simulink model "Testbench_for_Power_Circulating_TopologyB"  (R2023b)
settings: Solver=VariableStepAuto  StartTime=0.0  StopTime=1  RelTol=1e-3
InitFcn:
  | Initialization_for_Testbench;
values from neighbouring files (symbols this model uses):
  Cdc = 180e-6    (= 0.00018)    [CurrentLoop.m]    (also in Initialization_for_ESS_3P_2L_220kW.m; Initialization_for_Testbench.m)
  Fnom_Grid = 50    [CurrentLoop.m]    (also in Initialization_for_ESS_3P_2L_220kW.m; Initialization_for_Testbench.m)
  Inom = Pnom/sqrt(3)/Unom_Grid    [CurrentLoop.m]    (also in Initialization_for_ESS_3P_2L_220kW.m; Initialization_for_Testbench.m)
  Ki_Idq = Kp_Idq*2*pi*2    (= 40.2123859659)    [Initialization_for_ESS_3P_2L_220kW.m]    (also in Initialization_for_Testbench.m = 1.26330936334)
  Kp_Idq = L_grid/3/Ts_Control*3    (= 3.2)    [Initialization_for_ESS_3P_2L_220kW.m]    (also in Initialization_for_Testbench.m = 2.0106192983)
  L_grid = 200e-6    (= 0.0002)    [Initialization_for_ESS_3P_2L_220kW.m]    (also in Initialization_for_Testbench.m)
  Pnom = 220e3    (= 220000)    [CurrentLoop.m]    (also in Initialization_for_ESS_3P_2L_220kW.m; Initialization_for_Testbench.m = 2500000)
  Ts_Control = 62.5e-6    (= 6.25e-05)    [CurrentLoop.m]    (also in Initialization_for_ESS_3P_2L_220kW.m; Initialization_for_Testbench.m = 0.0001)
  Ts_Power = 10e-7    (= 1e-06)    [Initialization_for_ESS_3P_2L_220kW.m]    (also in Initialization_for_Testbench.m)
  Udc_ref = 1500    [CurrentLoop.m]    (also in Initialization_for_ESS_3P_2L_220kW.m; Initialization_for_Testbench.m)
  Unom_Phase = Unom_Grid/sqrt(3)    [CurrentLoop.m]    (also in Initialization_for_ESS_3P_2L_220kW.m; Initialization_for_Testbench.m)
libraries: LibraryForCodeGeneration x10, spsSeriesRLCBranchLib x4, spsTriangleGeneratorLib x2, spsUniversalBridgeLib x2, spsCurrentMeasurementLib x1, spsDCVoltageSourceLib x1, spsStairGeneratorLib x1, spsThreePhaseSeriesRLCBranchLib x1, spsThreePhaseVIMeasurementLib x1, spsVoltageMeasurementLib x1, spspowerguiLib x1
settings Model: DataDictionary=VariablesDictionary_for_Testbench_TopologyB.sldd  Creator=ZZY  LastModifiedBy=ZZY

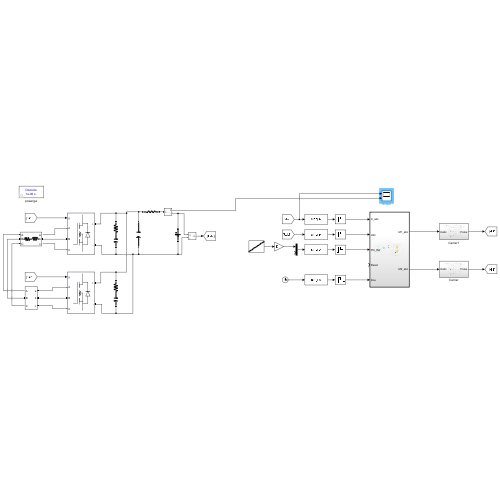
[thumbnail: Simulink's stored preview of the top-level diagram]
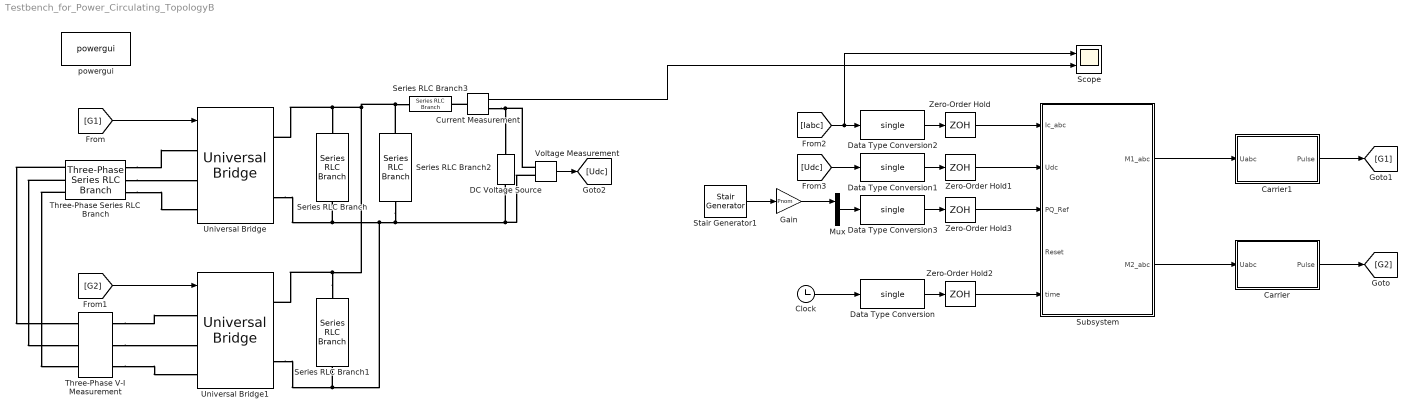
== system Testbench_for_Power_Circulating_TopologyB ==
  Carrier : Subsystem
  Carrier1 : Subsystem
  Clock : Clock
  Current Measurement : spsCurrentMeasurementLib/Current Measurement  PhasorSimulation=off  OutputType=Complex  PSBequivalent=0
  DC Voltage Source : spsDCVoltageSourceLib/DC Voltage Source  Amplitude=Udc_ref  Measurements=None
  Data Type Conversion{,1..3} (4 alike) : DataTypeConversion  OutDataTypeStr=single  SaturateOnIntegerOverflow=off  RndMeth=Floor
  Gain : Gain  Gain=Pnom
  Mux : Mux  Inputs=2
  Scope : Scope  NumInputPorts=2
  Series RLC Branch : spsSeriesRLCBranchLib/Series RLC Branch  LConnTagsString=__new0  RConnTagsString=__new0  BranchType=RC  Resistance=1e-6  Inductance=1e-3  SetiL0=off  InitialCurrent=0  Capacitance=Cdc  Setx0=on  InitialVoltage=Udc_ref  Measurements=Branch voltage
  Series RLC Branch1 : spsSeriesRLCBranchLib/Series RLC Branch  LConnTagsString=__new0  RConnTagsString=__new0  BranchType=RC  Resistance=1e-6  Inductance=1e-3  SetiL0=off  InitialCurrent=0  Capacitance=Cdc  Setx0=on  InitialVoltage=Udc_ref  Measurements=Branch voltage
  Series RLC Branch2 : spsSeriesRLCBranchLib/Series RLC Branch  LConnTagsString=__new0  RConnTagsString=__new0  BranchType=C  Resistance=1e-6  Inductance=1e-3  SetiL0=off  InitialCurrent=0  Capacitance=Cdc*100  Setx0=on  InitialVoltage=Udc_ref  Measurements=Branch voltage
  Series RLC Branch3 : spsSeriesRLCBranchLib/Series RLC Branch  LConnTagsString=__new0  RConnTagsString=__new0  BranchType=R  Resistance=1e-2  Inductance=1e-3  SetiL0=off  InitialCurrent=0  Capacitance=Cdc*100  Setx0=on  InitialVoltage=Udc_ref  Measurements=Branch voltage
  Stair Generator1 : spsStairGeneratorLib/Stair Generator  t=0:0.1:1  e=0:0.1:1  Ts=0
  Subsystem : Subsystem  TreatAsAtomicUnit=on  SystemSampleTime=Ts_Control
  Three-Phase Series RLC Branch : spsThreePhaseSeriesRLCBranchLib/Three-Phase Series RLC Branch  LConnTagsString=A|B|C  RConnTagsString=A|B|C  BranchType=RL  Resistance=1e-3  Inductance=L_grid*1  Capacitance=1e-6  Measurements=None
  Three-Phase V-I Measurement : spsThreePhaseVIMeasurementLib/Three-Phase V-I Measurement  VoltageMeasurement=no  SetLabelV=off  LabelV=Vabc  Vpu=off  VpuLL=off  CurrentMeasurement=yes  SetLabelI=on  LabelI=Iabc  Ipu=off  Pbase=100e6  Vbase=500e3  OutputType=Complex  PhasorSimulation=off  PSBequivalent=0
  Universal Bridge : spsUniversalBridgeLib/Universal Bridge  Arms=3  SnubberResistance=1e5  SnubberCapacitance=inf  Device=MOSFET / Diodes  Ron=1e-3  Lon=0  ForwardVoltages="[  0  0  ]"  ForwardVoltage=0  GTOparameters=[ 10e-6 , 20e-6 ]  IGBTparameters=[ 1e-6 , 2e-6 ]  Measurements=None  Measurements_2=None  converterType=Rectifier
  Universal Bridge1 : spsUniversalBridgeLib/Universal Bridge  Arms=3  SnubberResistance=1e5  SnubberCapacitance=inf  Device=MOSFET / Diodes  Ron=1e-3  Lon=0  ForwardVoltages="[  0  0  ]"  ForwardVoltage=0  GTOparameters=[ 10e-6 , 20e-6 ]  IGBTparameters=[ 1e-6 , 2e-6 ]  Measurements=None  Measurements_2=None  converterType=Rectifier
  Voltage Measurement : spsVoltageMeasurementLib/Voltage Measurement  PhasorSimulation=off  OutputType=Complex  PSBequivalent=0
  Zero-Order Hold{,1..3} (4 alike) : ZeroOrderHold  SampleTime=Ts_Control
  powergui : spspowerguiLib/powergui  Priority=1  SimulationMode=Discrete  SampleTime=Ts_Power  frequency=60  Iterations=50  frequencyindice=0  Pbase=100e6  ErrMax=1e-4  UnitsV=kV  UnitsW=MW  buscounter=0  FunctionMessages=off  echomessages=off  EnableUseOfTLC=off  CurrentSourceSwitches=off  DisableSnubberDevices=off  DisableRonSwitches=off  DisableVfSwitches=off  DisplayEquations=off  AutomaticDiscreteSolvers=off  SolverType=Tustin/Backward Euler (TBE)  Interpol=off  ExternalGateDelay=off  methode=off  Ts=100  x0status=blocks  SPID=on  SwTol=0  HookPort=off  NonlinearTolerance=1e-4  nMaxIteration=100  ContinueOnMaxIteration=off  RestoreLinks=warning  ResistiveCurrentMeasurement=off  Frange=[0:2:500]  Ylog=off  Xlog=on  ShowGrid=off  save=off  variable=ZData  structure=CHB_abc  ZoomFFT=off  StartTime=1.4  cycles=5  DisplayStyle=1  fundamental=50  FreqAxis=off  MaxFrequency=30000  frequencyindicesteady=1  RmsSteady=1  display=off
  wires:
  Subsystem/2(M2_abc) -> Carrier/1(Uabc)
  Carrier/1(Pulse) -> [G2]
  Carrier1/1(Pulse) -> [G1]
  Subsystem/1(M1_abc) -> Carrier1/1(Uabc)
  [G1] -> Universal Bridge/1
  [Iabc] -> Scope/1, Data Type Conversion2/1
  [G2] -> Universal Bridge1/1
  Zero-Order Hold/1 -> Subsystem/1(Ic_abc)
  Voltage Measurement/1 -> [Udc]
  [Udc] -> Data Type Conversion1/1
  Zero-Order Hold1/1 -> Subsystem/2(Udc)
  Clock/1 -> Data Type Conversion/1
  Zero-Order Hold2/1 -> Subsystem/5(time)
  Data Type Conversion/1 -> Zero-Order Hold2/1
  Data Type Conversion1/1 -> Zero-Order Hold1/1
  Data Type Conversion2/1 -> Zero-Order Hold/1
  Data Type Conversion3/1 -> Zero-Order Hold3/1
  Zero-Order Hold3/1 -> Subsystem/3(PQ_Ref)
  Mux/1 -> Data Type Conversion3/1
  Stair Generator1/1 -> Gain/1
  Gain/1 -> Mux/1
  Current Measurement/1 -> Scope/2
  connections:
  Series RLC Branch1/LConn1 -- Series RLC Branch3/RConn1 -- Series RLC Branch2/LConn1 -- Universal Bridge/RConn1 -- Series RLC Branch/LConn1 -- Universal Bridge1/RConn1
  Series RLC Branch1/RConn1 -- Voltage Measurement/LConn2 -- DC Voltage Source/LConn1 -- Series RLC Branch2/RConn1 -- Universal Bridge/RConn2 -- Series RLC Branch/RConn1 -- Universal Bridge1/RConn2
  Three-Phase Series RLC Branch/RConn2 -- Universal Bridge/LConn2
  Three-Phase Series RLC Branch/RConn1 -- Universal Bridge/LConn1
  Three-Phase Series RLC Branch/RConn3 -- Universal Bridge/LConn3
  Three-Phase Series RLC Branch/LConn3 -- Three-Phase V-I Measurement/LConn3
  Three-Phase Series RLC Branch/LConn2 -- Three-Phase V-I Measurement/LConn2
  Three-Phase Series RLC Branch/LConn1 -- Three-Phase V-I Measurement/LConn1
  Three-Phase V-I Measurement/RConn1 -- Universal Bridge1/LConn1
  Three-Phase V-I Measurement/RConn2 -- Universal Bridge1/LConn2
  Three-Phase V-I Measurement/RConn3 -- Universal Bridge1/LConn3
  Voltage Measurement/LConn1 -- Current Measurement/RConn1 -- DC Voltage Source/RConn1
  Current Measurement/LConn1 -- Series RLC Branch3/LConn1

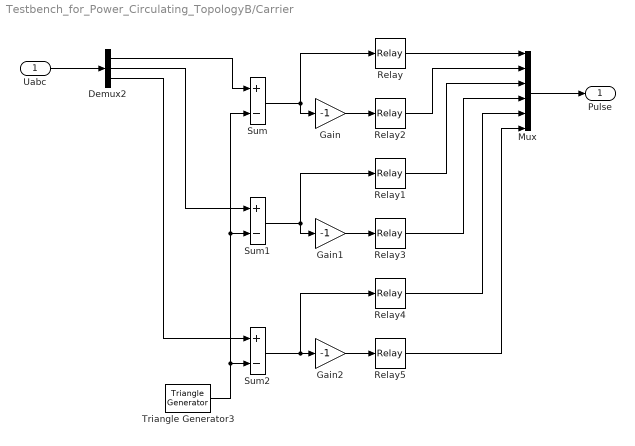
== system Testbench_for_Power_Circulating_TopologyB/Carrier ==
  Uabc : Inport
  Demux2 : Demux  Outputs=3
  Gain : Gain  Gain=-1
  Gain1 : Gain  Gain=-1
  Gain2 : Gain  Gain=-1
  Mux : Mux  Inputs=6
  Relay{,1..5} (6 alike) : Relay  OffSwitchValue=-eps
  Sum : Sum  Inputs=+-
  Sum1 : Sum  Inputs=+-
  Sum2 : Sum  Inputs=+-
  Triangle Generator3 : spsTriangleGeneratorLib/Triangle Generator  Freq=Fsw  Phase=180  Ts=Ts_Power
  Pulse : Outport
  wires:
  Mux/1 -> Pulse/1
  Gain/1 -> Relay2/1
  Sum/1 -> Relay/1, Gain/1
  Uabc/1 -> Demux2/1
  Demux2/1 -> Sum/1
  Relay/1 -> Mux/1
  Relay2/1 -> Mux/2
  Relay1/1 -> Mux/3
  Relay3/1 -> Mux/4
  Gain1/1 -> Relay3/1
  Demux2/2 -> Sum1/1
  Sum1/1 -> Relay1/1, Gain1/1
  Relay5/1 -> Mux/6
  Demux2/3 -> Sum2/1
  Gain2/1 -> Relay5/1
  Sum2/1 -> Relay4/1, Gain2/1
  Relay4/1 -> Mux/5
  Triangle Generator3/1 -> Sum/2, Sum1/2, Sum2/2

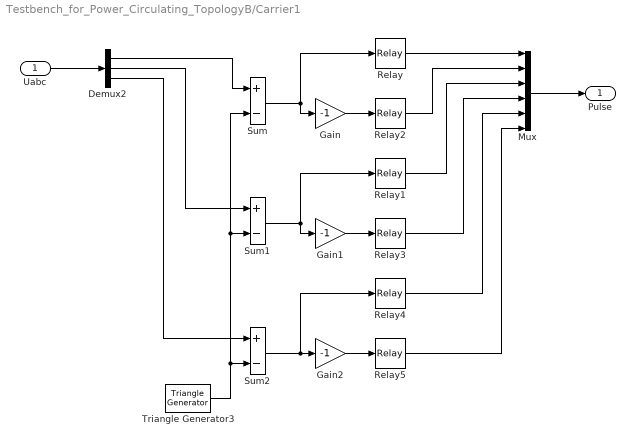
== system Testbench_for_Power_Circulating_TopologyB/Carrier1 ==
  Uabc : Inport
  Demux2 : Demux  Outputs=3
  Gain : Gain  Gain=-1
  Gain1 : Gain  Gain=-1
  Gain2 : Gain  Gain=-1
  Mux : Mux  Inputs=6
  Relay{,1..5} (6 alike) : Relay  OffSwitchValue=-eps
  Sum : Sum  Inputs=+-
  Sum1 : Sum  Inputs=+-
  Sum2 : Sum  Inputs=+-
  Triangle Generator3 : spsTriangleGeneratorLib/Triangle Generator  Freq=Fsw  Phase=180  Ts=Ts_Power
  Pulse : Outport
  wires:
  Mux/1 -> Pulse/1
  Gain/1 -> Relay2/1
  Sum/1 -> Relay/1, Gain/1
  Uabc/1 -> Demux2/1
  Demux2/1 -> Sum/1
  Relay/1 -> Mux/1
  Relay2/1 -> Mux/2
  Relay1/1 -> Mux/3
  Relay3/1 -> Mux/4
  Gain1/1 -> Relay3/1
  Demux2/2 -> Sum1/1
  Sum1/1 -> Relay1/1, Gain1/1
  Relay5/1 -> Mux/6
  Demux2/3 -> Sum2/1
  Gain2/1 -> Relay5/1
  Sum2/1 -> Relay4/1, Gain2/1
  Relay4/1 -> Mux/5
  Triangle Generator3/1 -> Sum/2, Sum1/2, Sum2/2

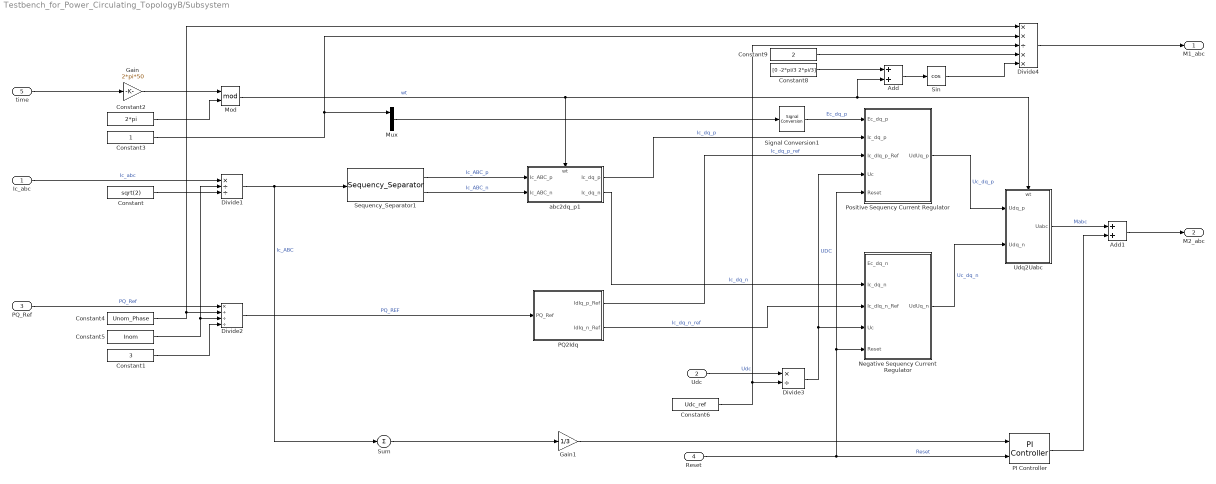
== system Testbench_for_Power_Circulating_TopologyB/Subsystem ==
  Ic_abc : Inport  OutDataTypeStr=single
  Udc : Inport  Port=2  OutDataTypeStr=single
  PQ_Ref : Inport  Port=3  OutDataTypeStr=single
  Reset : Inport  Port=4  OutDataTypeStr=boolean
  time : Inport  Port=5  OutDataTypeStr=single
  Add : Sum
  Add1 : Sum
  Constant : Constant  Value=sqrt(2)  OutDataTypeStr=single  SampleTime=-1
  Constant1 : Constant  Value=3  OutDataTypeStr=Inherit: Inherit via back propagation  SampleTime=-1
  Constant2 : Constant  Value=2*pi  OutDataTypeStr=single  SampleTime=-1
  Constant3 : Constant  OutDataTypeStr=single  SampleTime=-1
  Constant4 : Constant  Value=Unom_Phase  OutDataTypeStr=Inherit: Inherit via back propagation  SampleTime=-1
  Constant5 : Constant  Value=Inom  OutDataTypeStr=Inherit: Inherit via back propagation  SampleTime=-1
  Constant6 : Constant  Value=Udc_ref  OutDataTypeStr=Inherit: Inherit via back propagation  SampleTime=-1
  Constant8 : Constant  Value=[0 -2*pi/3 2*pi/3]  OutDataTypeStr=Inherit: Inherit via back propagation  SampleTime=-1
  Constant9 : Constant  Value=2  OutDataTypeStr=Inherit: Inherit via back propagation  SampleTime=-1
  Divide1 : Product  Inputs=*//  OutDataTypeStr=single
  Divide2 : Product  Inputs=*///  OutDataTypeStr=single
  Divide3 : Product  Inputs=*/  OutDataTypeStr=single
  Divide4 : Product  Inputs=**/**  OutDataTypeStr=single
  Gain : Gain  Gain=2*pi*50
  Gain1 : Gain  Gain=1/3
  Mod : Math  Operator=mod
  Mux : Mux  Inputs=2
  Negative Sequency Current Regulator : Subsystem
  PI Controller : LibraryForCodeGeneration/PI Controller  Kp=1  Ki=0.01  Ts=Ts_Control  Max=2  Min=-2
  PQ2Idq : Subsystem
  Positive Sequency Current Regulator : Subsystem
  Sequency_Separator1 : LibraryForCodeGeneration/Sequency_Separator  SystemSampleTime=-1  VariantActivationTime=update diagram  AllowFlexibleInterface=on  Latency=0  AutoFrameSizeCalculation=off
  Signal Conversion1 : SignalConversion  OverrideOpt=off
  Sin : Trigonometry  Operator=cos
  Sum : Sum  Inputs=+
  Udq2Uabc : Subsystem
      settings: PortSchema="{\"entries\":[{\"content\":{\"sides\":[{\"content\":{\"connectorIds\":[\"In1\",\"In2\"]},\"type\":\"ConnectorPlacement.EquallySpacedRectSide\",\"uuid\":\"009786f4-728c-4160-b9bf-eaf0b5a05101\"},{\"content\":{\"connectorIds\":[\"Out1\"],\"side\":\"RIGHT\"},\"type\":\"ConnectorPlacement.EquallySpacedRectSide\",\"uuid\":\"2a94367a-5c57-4632-9573-ab089470159a\"},{\"content\":{\"connectorIds\":[\"In3\"],\"side\":\"TOP\"},\"type\":\"ConnectorPlacement.EquallySpacedRectSide\",\"uuid\":\"6906365b-3187-4c4b-97cf-c9dec4c5ef7c\"}]},\"type\":\"ConnectorPlacement.EquallySpacedConnector\",\"uuid\":\"96ca8566-a266-405c-817a-b47b433d51ed\"}],\"packageUris\":[\"http://schema.mathworks.com/mf0/Connector/R2020b\"],\"version\":\"1.0\"}"
  abc2dq_p1 : Subsystem
      settings: PortSchema="{\"entries\":[{\"content\":{\"sides\":[{\"content\":{\"connectorIds\":[\"In1\",\"In2\"]},\"type\":\"ConnectorPlacement.EquallySpacedRectSide\",\"uuid\":\"702c7fae-dbbb-427d-af19-afd468018ae6\"},{\"content\":{\"connectorIds\":[\"Out1\",\"Out2\"],\"side\":\"RIGHT\"},\"type\":\"ConnectorPlacement.EquallySpacedRectSide\",\"uuid\":\"d2ca5462-a446-46d8-bb73-1a455ffa959f\"},{\"content\":{\"connectorIds\":[\"In3\"],\"side\":\"TOP\"},\"type\":\"ConnectorPlacement.EquallySpacedRectSide\",\"uuid\":\"50bc6c44-424f-4342-960e-11540364fe97\"}]},\"type\":\"ConnectorPlacement.EquallySpacedConnector\",\"uuid\":\"f58cf64d-fe35-43f1-a031-7ee625a8bb1e\"}],\"packageUris\":[\"http://schema.mathworks.com/mf0/Connector/R2020b\"],\"version\":\"1.0\"}"
  M1_abc : Outport  OutDataTypeStr=single
  M2_abc : Outport  Port=2  OutDataTypeStr=single
  wires:
  abc2dq_p1/2(Ic_dq_n) -> Negative Sequency Current Regulator/2(Ic_dq_n)  "Ic_dq_n"
  Udq2Uabc/1(Uabc) -> Add1/1  "Mabc"
  Mux/1 -> Signal Conversion1/1
  PQ2Idq/1(IdIq_p_Ref) -> Positive Sequency Current Regulator/3(Ic_dIq_p_Ref)  "Ic_dq_p_ref"
  Divide1/1 -> Sum/1, Sequency_Separator1/1  "Ic_ABC"
  Sequency_Separator1/2 -> abc2dq_p1/2("Ic_ABC_n ")  "Ic_ABC_n"
  PQ2Idq/2(IdIq_n_Ref) -> Negative Sequency Current Regulator/3(Ic_dIq_n_Ref)  "Ic_dq_n_ref"
  Sequency_Separator1/1 -> abc2dq_p1/1("Ic_ABC_p ")  "Ic_ABC_p"
  Constant4/1 -> Divide4/1, Divide2/2
  Constant5/1 -> Divide1/2, Divide2/3
  Reset/1 -> PI Controller/2, Positive Sequency Current Regulator/5(Reset), Negative Sequency Current Regulator/5(Reset)  "Reset"
  Constant6/1 -> Divide4/3, Divide3/2
  Negative Sequency Current Regulator/1(UdUq_n) -> Udq2Uabc/2(Udq_n)  "Uc_dq_n"
  Positive Sequency Current Regulator/1(UdUq_p) -> Udq2Uabc/1(Udq_p)  "Uc_dq_p"
  Divide3/1 -> Positive Sequency Current Regulator/4(Uc), Negative Sequency Current Regulator/4(Uc)  "UDC"
  Divide2/1 -> PQ2Idq/1(PQ_Ref)  "PQ_REF"
  Udc/1 -> Divide3/1  "Udc"
  Constant1/1 -> Divide2/4
  Mod/1 -> abc2dq_p1/3(wt), Add/2, Udq2Uabc/3(wt)  "wt"
  Ic_abc/1 -> Divide1/1  "Ic_abc"
  Constant/1 -> Divide1/3
  abc2dq_p1/1(Ic_dq_p) -> Positive Sequency Current Regulator/2(Ic_dq_p)  "Ic_dq_p"
  PQ_Ref/1 -> Divide2/1  "PQ_Ref"
  Constant2/1 -> Mod/2
  Constant3/1 -> Divide4/2, Mux/1
  Add/1 -> Sin/1
  Constant8/1 -> Add/1
  Divide4/1 -> M1_abc/1
  Sin/1 -> Divide4/5
  Constant9/1 -> Divide4/4
  time/1 -> Gain/1
  Gain/1 -> Mod/1
  Sum/1 -> Gain1/1
  Add1/1 -> M2_abc/1
  PI Controller/1 -> Add1/2
  Gain1/1 -> PI Controller/1
  Signal Conversion1/1 -> Positive Sequency Current Regulator/1(Ec_dq_p)  "Ec_dq_p"

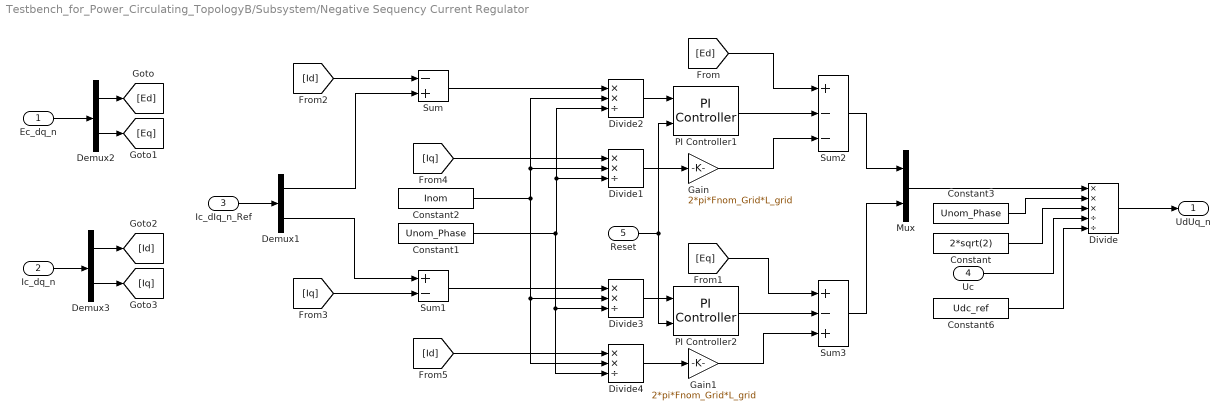
== system Testbench_for_Power_Circulating_TopologyB/Subsystem/Negative Sequency Current Regulator ==
  Ec_dq_n : Inport
  Ic_dq_n : Inport  Port=2
  Ic_dIq_n_Ref : Inport  Port=3
  Uc : Inport  Port=4
  Reset : Inport  Port=5  OutDataTypeStr=boolean
  Constant : Constant  Value=2*sqrt(2)  OutDataTypeStr=Inherit: Inherit via back propagation  SampleTime=-1
  Constant1 : Constant  Value=Unom_Phase  OutDataTypeStr=Inherit: Inherit via back propagation  SampleTime=-1
  Constant2 : Constant  Value=Inom  OutDataTypeStr=Inherit: Inherit via back propagation  SampleTime=-1
  Constant3 : Constant  Value=Unom_Phase  OutDataTypeStr=Inherit: Inherit via back propagation  SampleTime=-1
  Constant6 : Constant  Value=Udc_ref  OutDataTypeStr=Inherit: Inherit via back propagation  SampleTime=-1
  Demux1 : Demux  Outputs=2
  Demux2 : Demux  Outputs=2
  Demux3 : Demux  Outputs=2
  Divide : Product  Inputs=***//  OutDataTypeStr=single
  Divide{1..4} (4 alike) : Product  Inputs=**/  OutDataTypeStr=single
  Gain : Gain  Gain=2*pi*Fnom_Grid*L_grid  ParamDataTypeStr=Inherit: Same as input
  Gain1 : Gain  Gain=2*pi*Fnom_Grid*L_grid  ParamDataTypeStr=Inherit: Same as input
  Mux : Mux  Inputs=2
  PI Controller1 : LibraryForCodeGeneration/PI Controller  Kp=Kp_Idq  Ki=Ki_Idq  Ts=Ts_Control  Max=2  Min=-2
  PI Controller2 : LibraryForCodeGeneration/PI Controller  Kp=Kp_Idq  Ki=Ki_Idq  Ts=Ts_Control  Max=2  Min=-2
  Sum : Sum  Inputs=-+  InputSameDT=on  SaturateOnIntegerOverflow=on  OutDataTypeStr=Inherit: Same as first input
  Sum1 : Sum  Inputs=+-  InputSameDT=on  SaturateOnIntegerOverflow=on  OutDataTypeStr=Inherit: Same as first input
  Sum2 : Sum  Inputs=+--  InputSameDT=on  SaturateOnIntegerOverflow=on  OutDataTypeStr=Inherit: Same as first input
  Sum3 : Sum  Inputs=+-+  InputSameDT=on  SaturateOnIntegerOverflow=on  OutDataTypeStr=Inherit: Same as first input
  UdUq_n : Outport
  wires:
  [Id] -> Divide4/1
  [Iq] -> Divide1/1
  [Iq] -> Sum1/2
  [Id] -> Sum/1
  Ic_dq_n/1 -> Demux3/1
  Demux3/1 -> [Id]
  Demux3/2 -> [Iq]
  Demux1/2 -> Sum1/1
  Demux1/1 -> Sum/2
  [Eq] -> Sum3/1
  [Ed] -> Sum2/1
  Demux2/2 -> [Eq]
  Demux2/1 -> [Ed]
  Divide3/1 -> PI Controller2/1
  Sum/1 -> Divide2/1
  Mux/1 -> Divide/1
  Divide/1 -> UdUq_n/1
  Gain1/1 -> Sum3/3
  Gain/1 -> Sum2/3
  Ec_dq_n/1 -> Demux2/1
  Ic_dIq_n_Ref/1 -> Demux1/1
  Sum2/1 -> Mux/1
  Sum1/1 -> Divide3/1
  Divide2/1 -> PI Controller1/1
  Sum3/1 -> Mux/2
  Reset/1 -> PI Controller2/2, PI Controller1/2
  Constant3/1 -> Divide/2
  Constant/1 -> Divide/3
  Uc/1 -> Divide/4
  Constant6/1 -> Divide/5
  Divide1/1 -> Gain/1
  Divide4/1 -> Gain1/1
  Constant2/1 -> Divide1/2, Divide2/2, Divide4/2, Divide3/2
  Constant1/1 -> Divide3/3, Divide4/3, Divide1/3, Divide2/3
  PI Controller2/1 -> Sum3/2
  PI Controller1/1 -> Sum2/2

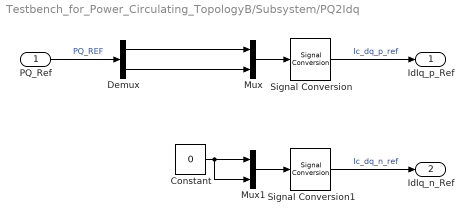
== system Testbench_for_Power_Circulating_TopologyB/Subsystem/PQ2Idq ==
  PQ_Ref : Inport
  Constant : Constant  Value=0  OutDataTypeStr=Inherit: Inherit via back propagation  SampleTime=-1
  Demux : Demux  Outputs=2
  Mux : Mux  Inputs=2
  Mux1 : Mux  Inputs=2
  Signal Conversion : SignalConversion  OverrideOpt=off
  Signal Conversion1 : SignalConversion  OverrideOpt=off
  IdIq_p_Ref : Outport
  IdIq_n_Ref : Outport  Port=2
  wires:
  Mux1/1 -> Signal Conversion1/1
  Mux/1 -> Signal Conversion/1
  PQ_Ref/1 -> Demux/1  "PQ_REF"
  Demux/2 -> Mux/2
  Demux/1 -> Mux/1
  Signal Conversion/1 -> IdIq_p_Ref/1  "Ic_dq_p_ref"
  Signal Conversion1/1 -> IdIq_n_Ref/1  "Ic_dq_n_ref"
  Constant/1 -> Mux1/2, Mux1/1

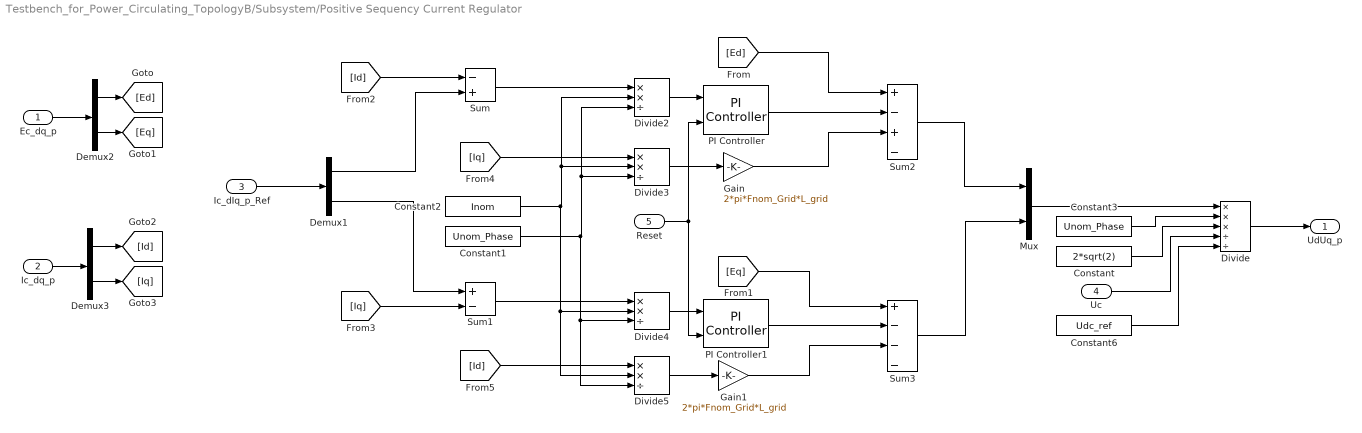
== system Testbench_for_Power_Circulating_TopologyB/Subsystem/Positive Sequency Current Regulator ==
  Ec_dq_p : Inport
  Ic_dq_p : Inport  Port=2
  Ic_dIq_p_Ref : Inport  Port=3
  Uc : Inport  Port=4
  Reset : Inport  Port=5  OutDataTypeStr=boolean
  Constant : Constant  Value=2*sqrt(2)  OutDataTypeStr=Inherit: Inherit via back propagation  SampleTime=-1
  Constant1 : Constant  Value=Unom_Phase  OutDataTypeStr=Inherit: Inherit via back propagation  SampleTime=-1
  Constant2 : Constant  Value=Inom  OutDataTypeStr=Inherit: Inherit via back propagation  SampleTime=-1
  Constant3 : Constant  Value=Unom_Phase  OutDataTypeStr=Inherit: Inherit via back propagation  SampleTime=-1
  Constant6 : Constant  Value=Udc_ref  OutDataTypeStr=Inherit: Inherit via back propagation  SampleTime=-1
  Demux1 : Demux  Outputs=2
  Demux2 : Demux  Outputs=2
  Demux3 : Demux  Outputs=2
  Divide : Product  Inputs=***//  OutDataTypeStr=single
  Divide{2..5} (4 alike) : Product  Inputs=**/  OutDataTypeStr=single
  Gain : Gain  Gain=2*pi*Fnom_Grid*L_grid  ParamDataTypeStr=Inherit: Same as input
  Gain1 : Gain  Gain=2*pi*Fnom_Grid*L_grid  ParamDataTypeStr=Inherit: Same as input
  Mux : Mux  Inputs=2
  PI Controller : LibraryForCodeGeneration/PI Controller  Kp=Kp_Idq  Ki=Ki_Idq  Ts=Ts_Control  Max=2  Min=-2
  PI Controller1 : LibraryForCodeGeneration/PI Controller  Kp=Kp_Idq  Ki=Ki_Idq  Ts=Ts_Control  Max=2  Min=-2
  Sum : Sum  Inputs=-+  InputSameDT=on  SaturateOnIntegerOverflow=on  OutDataTypeStr=Inherit: Same as first input
  Sum1 : Sum  Inputs=+-  InputSameDT=on  SaturateOnIntegerOverflow=on  OutDataTypeStr=Inherit: Same as first input
  Sum2 : Sum  Inputs=+-+-  InputSameDT=on  SaturateOnIntegerOverflow=on  OutDataTypeStr=Inherit: Same as first input
  Sum3 : Sum  Inputs=+---  InputSameDT=on  SaturateOnIntegerOverflow=on  OutDataTypeStr=Inherit: Same as first input
  UdUq_p : Outport
  wires:
  Sum3/1 -> Mux/2
  Sum1/1 -> Divide4/1
  Sum2/1 -> Mux/1
  Ic_dIq_p_Ref/1 -> Demux1/1
  Uc/1 -> Divide/4
  Divide3/1 -> Gain/1
  Divide5/1 -> Gain1/1
  Ec_dq_p/1 -> Demux2/1
  Gain/1 -> Sum2/3
  Divide/1 -> UdUq_p/1
  Mux/1 -> Divide/1
  Sum/1 -> Divide2/1
  Divide4/1 -> PI Controller1/1
  Demux2/1 -> [Ed]
  Demux2/2 -> [Eq]
  [Ed] -> Sum2/1
  Demux1/1 -> Sum/2
  Demux1/2 -> Sum1/1
  Demux3/2 -> [Iq]
  Demux3/1 -> [Id]
  Ic_dq_p/1 -> Demux3/1
  [Id] -> Sum/1
  [Iq] -> Sum1/2
  [Iq] -> Divide3/1
  [Id] -> Divide5/1
  PI Controller/1 -> Sum2/2
  Divide2/1 -> PI Controller/1
  Reset/1 -> PI Controller1/2, PI Controller/2
  Constant3/1 -> Divide/2
  Constant/1 -> Divide/3
  Constant6/1 -> Divide/5
  Constant2/1 -> Divide5/2, Divide4/2, Divide3/2, Divide2/2
  Constant1/1 -> Divide5/3, Divide4/3, Divide3/3, Divide2/3
  [Eq] -> Sum3/1
  PI Controller1/1 -> Sum3/2
  Gain1/1 -> Sum3/3

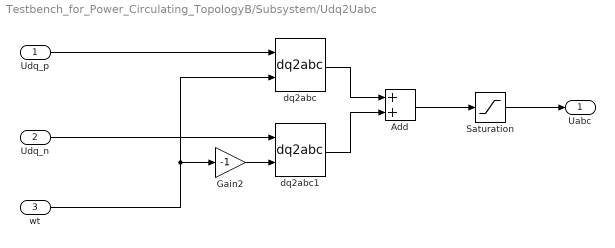
== system Testbench_for_Power_Circulating_TopologyB/Subsystem/Udq2Uabc ==
  Udq_p : Inport
  Udq_n : Inport  Port=2
  wt : Inport  Port=3
  Add : Sum
  Gain2 : Gain  Gain=-1  ParamDataTypeStr=Inherit: Same as input
  Saturation : Saturate  UpperLimit=1.15  LowerLimit=-1.15
  dq2abc : LibraryForCodeGeneration/dq2abc  SystemSampleTime=-1  VariantActivationTime=update diagram  AllowFlexibleInterface=on  Latency=0  AutoFrameSizeCalculation=off
  dq2abc1 : LibraryForCodeGeneration/dq2abc  SystemSampleTime=-1  VariantActivationTime=update diagram  AllowFlexibleInterface=on  Latency=0  AutoFrameSizeCalculation=off
  Uabc : Outport
  wires:
  dq2abc1/1 -> Add/2
  wt/1 -> dq2abc/2, Gain2/1
  Gain2/1 -> dq2abc1/2
  Udq_p/1 -> dq2abc/1
  Udq_n/1 -> dq2abc1/1
  Add/1 -> Saturation/1
  dq2abc/1 -> Add/1
  Saturation/1 -> Uabc/1

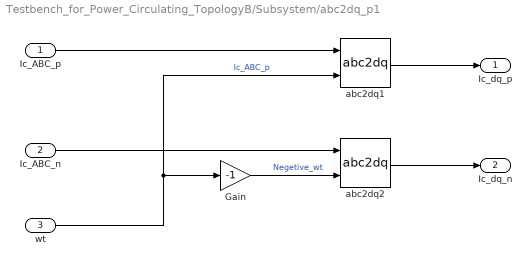
== system Testbench_for_Power_Circulating_TopologyB/Subsystem/abc2dq_p1 ==
  "Ic_ABC_p " : Inport
  "Ic_ABC_n " : Inport  Port=2
  wt : Inport  Port=3
  Gain : Gain  Gain=-1
  abc2dq1 : LibraryForCodeGeneration/abc2dq  SystemSampleTime=-1  VariantActivationTime=update diagram  AllowFlexibleInterface=on  Latency=0  AutoFrameSizeCalculation=off
  abc2dq2 : LibraryForCodeGeneration/abc2dq  SystemSampleTime=-1  VariantActivationTime=update diagram  AllowFlexibleInterface=on  Latency=0  AutoFrameSizeCalculation=off
  Ic_dq_p : Outport
  Ic_dq_n : Outport  Port=2
  wires:
  "Ic_ABC_p "/1 -> abc2dq1/1
  abc2dq1/1 -> Ic_dq_p/1
  Gain/1 -> abc2dq2/2  "Negetive_wt"
  "Ic_ABC_n "/1 -> abc2dq2/1
  abc2dq2/1 -> Ic_dq_n/1
  wt/1 -> abc2dq1/2, Gain/1  "Ic_ABC_p"
